simulink model "adjcochanint"  (Simulink 6.0)
settings: Solver=VariableStepDiscrete  SolverMode=SingleTasking  StartTime=0.0  StopTime=50000  RelTol=1e-3  AbsTol=1e-6
undefined symbols (not defined in the file or in its folder): Fs, Rows, slcm, Tsym
libraries: dspsrcs4 x8, simulink x5, commdigbbndpm2 x4, dspsigattribs x4, commfilt2 x4, commrandsrc2 x3, commsink2 x2, dspsnks4 x2, dspmathops x2, commchan2 x1, dspsigops x1
CloseFcn:
  | clear adjcoSigsOut
settings Model: RequirementInfo=9  CovMetricSettings=d  Creator=tdelve  LastModifiedBy=arodrigu  ExtModeTrigMode=oneshot  ExtModeArmWhenConnect=off  ExtModeAutoUpdateStatusClock=off  ProdHWDeviceType=Specified
settings DataIOCC: LimitDataPoints=off  SaveOutput=off  SaveTime=off  SignalLoggingName=adjcoSigsOut
settings OptimizationCC: BlockReduction=off  BooleanDataType=off
settings DebuggingCC: CheckExecutionContextPreStartOutputMsg=on  CheckExecutionContextRuntimeOutputMsg=on  SolverPrmCheckMsg=none  InheritedTsInSrcMsg=none  IntegerOverflowMsg=none
settings HardwareCC: ProdHWDeviceType=Specified
settings ModelReferenceCC: UpdateModelReferenceTargets=IfOutOfDate
settings CodeAppCC: MangleLength=5

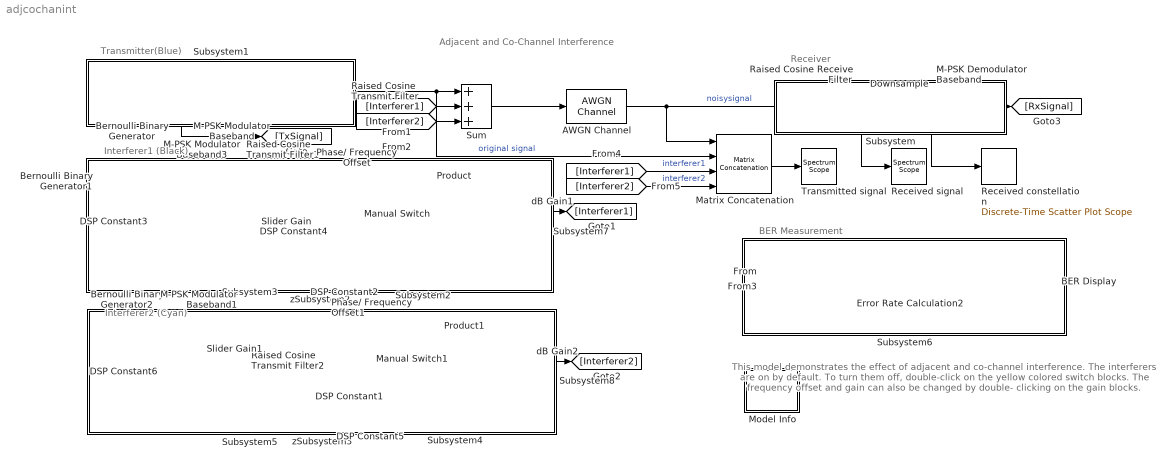
== system adjcochanint ==
  note: Adjacent and Co-Channel Interference
  note: Interferer1 (Black)
  note: Transmitter(Blue)
  note: Interferer2 (Cyan)
  note: Receiver
  note: BER Measurement
  note: This model demonstrates the effect of adjacent
      | and co-channel interference. The interferers are
      | on by default. To turn them off, double-click on
      | the yellow colored switch blocks. The frequency
      | offset and gain can also be changed by double-
      | clicking on the gain blocks.
  AWGN Channel : commchan2/AWGN Channel  seed=123456  noiseMode="Signal to noise ratio  (Es/No)"  EbNodB=10  EsNodB=30  SNRdB=10  bitsPerSym=1  Ps=1/8  Tsym=1e-6  variance=1
  BER Display : Display
  Bernoulli Binary Generator : commrandsrc2/Bernoulli Binary Generator  P=0.5  seed=529558  Ts=1e-6/3  frameBased=on  sampPerFrame=300  orient=off
  Bernoulli Binary Generator1 : commrandsrc2/Bernoulli Binary Generator  P=0.5  seed=529573  Ts=1e-6/3  frameBased=on  sampPerFrame=300  orient=off
  Bernoulli Binary Generator2 : commrandsrc2/Bernoulli Binary Generator  P=0.5  seed=529397  Ts=1e-6/3  frameBased=on  sampPerFrame=300  orient=off
  DSP Constant1 : dspsrcs4/DSP Constant  Value=0  SampleMode=Discrete  discreteOutput=Frame-based  continuousOutput=Sample-based  sampTime=Tsym*300  framePeriod=(1e-6/3)*300  dataType=Inherit from 'Constant value'  isSigned=on  wordLen=16  udDataType=sfix(16)  fracBitsMode=Best precision  numFracBits=15  InterpretAs1D=-inf  Ts=-inf  FramebasedOutput=-inf
  DSP Constant2 : dspsrcs4/DSP Constant  Value=1  SampleMode=Discrete  discreteOutput=Frame-based  continuousOutput=Sample-based  sampTime=Tsym*300  framePeriod=(1e-6/3)*300  dataType=Inherit from 'Constant value'  isSigned=on  wordLen=16  udDataType=sfix(16)  fracBitsMode=Best precision  numFracBits=15  InterpretAs1D=-inf  Ts=-inf  FramebasedOutput=-inf
  DSP Constant3 : dspsrcs4/DSP Constant  Value=-4e6  SampleMode=Discrete  discreteOutput=Frame-based  continuousOutput=Sample-based  sampTime=Tsym*100  framePeriod=(1e-6/3)*300  dataType=Inherit from 'Constant value'  isSigned=on  wordLen=16  udDataType=sfix(16)  fracBitsMode=Best precision  numFracBits=15  InterpretAs1D=-inf  Ts=-inf  FramebasedOutput=-inf
  DSP Constant4 : dspsrcs4/DSP Constant  Value=0  SampleMode=Discrete  discreteOutput=Frame-based  continuousOutput=Sample-based  sampTime=Tsym*300  framePeriod=(1e-6/3)*300  dataType=Inherit from 'Constant value'  isSigned=on  wordLen=16  udDataType=sfix(16)  fracBitsMode=Best precision  numFracBits=15  InterpretAs1D=-inf  Ts=-inf  FramebasedOutput=-inf
  DSP Constant5 : dspsrcs4/DSP Constant  Value=1  SampleMode=Discrete  discreteOutput=Frame-based  continuousOutput=Sample-based  sampTime=Tsym*300  framePeriod=(1e-6/3)*300  dataType=Inherit from 'Constant value'  isSigned=on  wordLen=16  udDataType=sfix(16)  fracBitsMode=Best precision  numFracBits=15  InterpretAs1D=-inf  Ts=-inf  FramebasedOutput=-inf
  DSP Constant6 : dspsrcs4/DSP Constant  Value=4e6  SampleMode=Discrete  discreteOutput=Frame-based  continuousOutput=Sample-based  sampTime=Tsym*300  framePeriod=(1e-6/3)*300  dataType=Inherit from 'Constant value'  isSigned=on  wordLen=16  udDataType=sfix(16)  fracBitsMode=Best precision  numFracBits=15  InterpretAs1D=-inf  Ts=-inf  FramebasedOutput=-inf
  Downsample : dspsigops/Downsample  N=8  phase=0  ic=0  smode=Allow multirate  fmode=Maintain input frame rate
  Error Rate Calculation2 : commsink2/Error Rate Calculation  N=12*3  st_delay=0  cp_mode=Entire frame  subframe=[]  PMode=Port  WsName=e1  RsMode2=off  stop=off  numErr=100  maxBits=1e6
  M-PSK Demodulator Baseband : commdigbbndpm2/M-PSK Demodulator Baseband  M=8  OutType=Bit  Dec=Gray  Ph=0  numSamp=1
  M-PSK Modulator Baseband : commdigbbndpm2/M-PSK Modulator Baseband  M=8  InType=Bit  Enc=Gray  Ph=0  numSamp=1
  M-PSK Modulator Baseband1 : commdigbbndpm2/M-PSK Modulator Baseband  M=8  InType=Bit  Enc=Gray  Ph=0  numSamp=1
  M-PSK Modulator Baseband3 : commdigbbndpm2/M-PSK Modulator Baseband  M=8  InType=Bit  Enc=Gray  Ph=0  numSamp=1
  Manual Switch : simulink/Signal Routing/Manual Switch  sw=0  action=0
  Manual Switch1 : simulink/Signal Routing/Manual Switch  sw=0  action=0
  Matrix Concatenation : simulink/Math Operations/Matrix Concatenation  numInports=4  catMethod=Horizontal
  Model Info : Subsystem  LoadFcn=slcm LoadBlock;  InitFcn=slcm('UpdateAllCMBlocksInThisModelInit')  PropExecContextAcrossSSBoundary=on  mask(CMBlock){InitialSaveTempField=, InitialBlockCM=none, BlockCM=none, Frame=on, SaveTempField=, DisplayStringWithTags=Info, MaskDisplayString=Info, HorizontalTextAlignment=Center, LeftAlignmentValue=0.5, SourceBlockDiagram=adjcochanint, TagMaxNumber=20, CMTag1=, CMTag2=, CMTag3=, CMTag4=, CMTag5=, CMTag6=, CMTag7=, CMTag8=, CMTag9=, CMTag10=, CMTag11=, CMTag12=, CMTag13=, CMTag14=, CMTag15=, CMTag16=, CMTag17=, CMTag18=, CMTag19=, CMTag20=}
      mask help: This block allows revision control information to be displayed within the model.
      settings: CopyFcn=slcm CopyBlock;  DeleteFcn=slcm Cancel;  PostSaveFcn=slcm('UpdateAllCMBlocksInThisModel')  NameChangeFcn=slcm Rename;  OpenFcn=commdemohelp;
      mask Display: text(str2num(LeftAlignmentValue), 0.5, MaskDisplayString, 'HorizontalAlignment', HorizontalTextAlignment)
  Phase/ Frequency Offset : Subsystem  PropExecContextAcrossSSBoundary=on  mask(Phase/Frequency Offset){phaseOffset=0}
      mask prompts: phaseOffset "Phase offset (deg):"
      mask help: Complex baseband model of residual phase and frequency offsets.
      mask Help: helpview(commbhelp)
      mask Display: disp('Phase/\nFrequency\nOffset');
  Phase/ Frequency Offset1 : Subsystem  PropExecContextAcrossSSBoundary=on  mask(Phase/Frequency Offset){phaseOffset=0}
      mask prompts: phaseOffset "Phase offset (deg):"
      mask help: Complex baseband model of residual phase and frequency offsets.
      mask Help: helpview(commbhelp)
      mask Display: disp('Phase/\nFrequency\nOffset');
  Product : Product  SaturateOnIntegerOverflow=on
  Product1 : Product  SaturateOnIntegerOverflow=on
  Raised Cosine Receive Filter : commfilt2/Raised Cosine Receive Filter  filtType=Square root  N=8  D=6  R=0.22  sampMode=Frame-based  rateMode=None  downFactor=1  downOffset=0  checkGain=Normalized  filterGain=1  checkCoeff=off  variableName=rcRxFilt  launchFVT=off
  Raised Cosine Transmit Filter : commfilt2/Raised Cosine Transmit Filter  filtType=Square root  D=6  R=0.22  sampMode=Frame-based  N=8  checkGain=Normalized  filterGain=1  checkCoeff=off  variableName=rcTxFilt  launchFVT=off
  Raised Cosine Transmit Filter1 : commfilt2/Raised Cosine Transmit Filter  filtType=Square root  D=6  R=0.22  sampMode=Frame-based  N=8  checkGain=Normalized  filterGain=1  checkCoeff=off  variableName=rcTxFilt1  launchFVT=off
  Raised Cosine Transmit Filter2 : commfilt2/Raised Cosine Transmit Filter  filtType=Square root  D=6  R=0.22  sampMode=Frame-based  N=8  checkGain=Normalized  filterGain=1  checkCoeff=off  variableName=rcTxFilt2  launchFVT=off
  Received constellation : commsink2/Discrete-Time Scatter Plot Scope  Tag=ScatterPlot  sampPerSymb=1  offsetEye=0  numTraces=400  numNewFrames=100  LineMarkers=.  LineColors=b  fading=on  render=on  AxisGrid=on  xMin=-2.4831480177732  xMax=2.52514227621423  yMin=-2.47259861231716  yMax=2.53569168167027  inphaseLabel=In-phase Amplitude  quadratureLabel=Quadrature Amplitude  openScopeAtSimStart=on  FrameNumber=off  FigPos=[788 34 211 211]  figTitle=Scatter Plot  numLinesMax=8  block_type_=scatter
  Received signal : dspsnks4/Spectrum Scope  ScopeProperties=off  Domain=Frequency  HorizSpan=1  UseBuffer=on  BufferSize=128  Overlap=64  inpFftLenInherit=off  FFTlength=128  numAvg=10  DisplayProperties=on  AxisGrid=on  Memory=off  FrameNumber=off  AxisLegend=off  AxisZoom=off  OpenScopeAtSimStart=on  OpenScopeImmediately=off  FigPos=[381 47 357 145]  AxisProperties=off  XUnits=Hertz  XRange=[-Fs/2...Fs/2]  InheritXIncr=on  XIncr=1.0  XLabel=Samples  YUnits=dB  YLabel=Magnitude, dB  LineProperties=off  LineColors=[1 0 0]|[0 0 1]
      settings: YMin=-95.9893424566119  YMax=19.7294255518364
  Slider Gain : simulink/Math Operations/Slider Gain  low=0  gain=1  high=2
  Slider Gain1 : simulink/Math Operations/Slider Gain  low=0  gain=1.4  high=2
  Subsystem : Subsystem  Orientation=left  PropExecContextAcrossSSBoundary=on
      mask Display: disp('');
  Subsystem1 : Subsystem  Orientation=left  PropExecContextAcrossSSBoundary=on
      mask Display: disp('');
  Subsystem2 : Subsystem  Orientation=left  PropExecContextAcrossSSBoundary=on
      mask Display: disp('Double-click above\n to activate Interferer1');
  Subsystem3 : Subsystem  Orientation=left  PropExecContextAcrossSSBoundary=on
      mask Display: disp('Double-click above\n to change frequency offset');
  Subsystem4 : Subsystem  Orientation=left  PropExecContextAcrossSSBoundary=on
      mask Display: disp('Double-click above\n to activate Interferer2');
  Subsystem5 : Subsystem  Orientation=left  PropExecContextAcrossSSBoundary=on
      mask Display: disp('Double-click above\n to change frequency offset');
  Subsystem6 : Subsystem  Orientation=left  PropExecContextAcrossSSBoundary=on
      mask Display: disp('');
  Subsystem7 : Subsystem  Orientation=left  PropExecContextAcrossSSBoundary=on
      mask Display: disp('Double-click above\n to change gain');
  Subsystem8 : Subsystem  Orientation=left  PropExecContextAcrossSSBoundary=on
      mask Display: disp('Double-click above\n to change gain');
  Sum : Sum  Inputs=+++  SaturateOnIntegerOverflow=on
  Transmitted signal : dspsnks4/Spectrum Scope  ScopeProperties=off  Domain=Frequency  HorizSpan=1  UseBuffer=on  BufferSize=128  Overlap=64  inpFftLenInherit=off  FFTlength=128  numAvg=10  DisplayProperties=on  AxisGrid=on  Memory=off  FrameNumber=off  AxisLegend=off  AxisZoom=off  OpenScopeAtSimStart=on  OpenScopeImmediately=off  FigPos=[10 47 357 145]  AxisProperties=off  XUnits=Hertz  XRange=[-Fs/2...Fs/2]  InheritXIncr=on  XIncr=1.0  XLabel=Samples  YUnits=dB  YLabel=Magnitude, dB  LineProperties=off  LineColors=[1 0 0]|[0 0 1]|[0 0 0]|[0 1 1]
      settings: YMin=-91.8082302358486  YMax=10.0230122396749
  dB Gain1 : dspmathops/dB Gain  dB=-20  intype=Amplitude
  dB Gain2 : dspmathops/dB Gain  dB=-10  intype=Amplitude
  zSubsystem2 : Subsystem  Orientation=left  PropExecContextAcrossSSBoundary=on
      mask Display: disp('');
  zSubsystem3 : Subsystem  Orientation=left  PropExecContextAcrossSSBoundary=on
      mask Display: disp('');
  wires:
  M-PSK Modulator Baseband/1 -> Raised Cosine Transmit Filter/1
  Bernoulli Binary Generator1/1 -> M-PSK Modulator Baseband3/1
  M-PSK Modulator Baseband1/1 -> Raised Cosine Transmit Filter2/1
  M-PSK Modulator Baseband3/1 -> Raised Cosine Transmit Filter1/1
  Raised Cosine Transmit Filter1/1 -> Phase/ Frequency Offset/1(In)
  Raised Cosine Transmit Filter2/1 -> Phase/ Frequency Offset1/1(In)
  Raised Cosine Transmit Filter/1 -> Sum/1, Matrix Concatenation/2  "original signal"
  DSP Constant4/1 -> Manual Switch/1
  Manual Switch/1 -> Product/2
  DSP Constant2/1 -> Manual Switch/2
  DSP Constant1/1 -> Manual Switch1/1
  Manual Switch1/1 -> Product1/2
  DSP Constant5/1 -> Manual Switch1/2
  Phase/ Frequency Offset1/1(Out) -> Product1/1
  Slider Gain/1 -> Phase/ Frequency Offset/2(In1)
  DSP Constant3/1 -> Slider Gain/1
  DSP Constant6/1 -> Slider Gain1/1
  Slider Gain1/1 -> Phase/ Frequency Offset1/2(In1)
  Bernoulli Binary Generator/1 -> M-PSK Modulator Baseband/1, [TxSignal]
  Bernoulli Binary Generator2/1 -> M-PSK Modulator Baseband1/1
  Phase/ Frequency Offset/1(Out) -> Product/1
  Sum/1 -> AWGN Channel/1
  AWGN Channel/1 -> Raised Cosine Receive Filter/1, Matrix Concatenation/1  "noisysignal"
  Raised Cosine Receive Filter/1 -> Received signal/1, Downsample/1
  Downsample/1 -> Received constellation/1, M-PSK Demodulator Baseband/1
  M-PSK Demodulator Baseband/1 -> [RxSignal]
  Product/1 -> dB Gain1/1
  Product1/1 -> dB Gain2/1
  [Interferer1] -> Sum/2
  [Interferer2] -> Sum/3
  Matrix Concatenation/1 -> Transmitted signal/1
  [TxSignal] -> Error Rate Calculation2/1
  [RxSignal] -> Error Rate Calculation2/2
  dB Gain1/1 -> [Interferer1]
  dB Gain2/1 -> [Interferer2]
  [Interferer1] -> Matrix Concatenation/3  "interferer1"
  [Interferer2] -> Matrix Concatenation/4  "interferer2"
  Error Rate Calculation2/1 -> BER Display/1

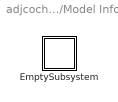
== system adjcochanint/Model Info ==
  EmptySubsystem : Subsystem  PropExecContextAcrossSSBoundary=on

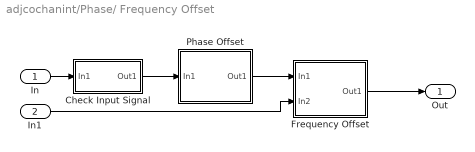
== system adjcochanint/Phase/ Frequency Offset ==
  In : Inport  LatchInput=off
  In1 : Inport  Port=2  LatchInput=off
  Check Input Signal : Subsystem  PropExecContextAcrossSSBoundary=on
      mask Display: disp('Check\nInput Signal');
  Frequency Offset : Subsystem  PropExecContextAcrossSSBoundary=on
      mask Display: disp('Frequency\nOffset');
  Phase Offset : Subsystem  PropExecContextAcrossSSBoundary=on
      mask Display: disp('Phase\nOffset');
  Out : Outport
  wires:
  Check Input Signal/1(Out1) -> Phase Offset/1(In1)
  Phase Offset/1(Out1) -> Frequency Offset/1(In1)
  In/1 -> Check Input Signal/1(In1)
  Frequency Offset/1(Out1) -> Out/1
  In1/1 -> Frequency Offset/2(In2)

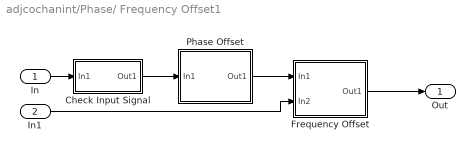
== system adjcochanint/Phase/ Frequency Offset1 ==
  In : Inport  LatchInput=off
  In1 : Inport  Port=2  LatchInput=off
  Check Input Signal : Subsystem  PropExecContextAcrossSSBoundary=on
      mask Display: disp('Check\nInput Signal');
  Frequency Offset : Subsystem  PropExecContextAcrossSSBoundary=on
      mask Display: disp('Frequency\nOffset');
  Phase Offset : Subsystem  PropExecContextAcrossSSBoundary=on
      mask Display: disp('Phase\nOffset');
  Out : Outport
  wires:
  In1/1 -> Frequency Offset/2(In2)
  Frequency Offset/1(Out1) -> Out/1
  In/1 -> Check Input Signal/1(In1)
  Phase Offset/1(Out1) -> Frequency Offset/1(In1)
  Check Input Signal/1(Out1) -> Phase Offset/1(In1)

== system adjcochanint/Subsystem ==

== system adjcochanint/Subsystem1 ==

== system adjcochanint/Subsystem2 ==

== system adjcochanint/Subsystem3 ==

== system adjcochanint/Subsystem4 ==

== system adjcochanint/Subsystem5 ==

== system adjcochanint/Subsystem6 ==

== system adjcochanint/Subsystem7 ==

== system adjcochanint/Subsystem8 ==

== system adjcochanint/zSubsystem2 ==

== system adjcochanint/zSubsystem3 ==

== system adjcochanint/Model Info/EmptySubsystem ==

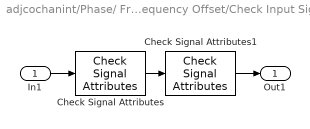
== system adjcochanint/Phase/ Frequency Offset/Check Input Signal ==
  In1 : Inport  LatchInput=off
  Check Signal Attributes : dspsigattribs/Check Signal Attributes  SigAttribCheckMethod=Does not match attributes exactly  Complexity=Complex  Frame=Ignore  DimsCheckMethod=Is...  Dimensions=Column vector (2-D) or scalar  DatatypeCheckMethod=Ignore  DatatypeGeneral=Boolean  DtypeFloatSpecific=Any floating-point  DtypeFixedSpecific=Any fixed-point  DtypeIntSpecific=Any integer  SampleMode=Ignore
  Check Signal Attributes1 : dspsigattribs/Check Signal Attributes  SigAttribCheckMethod=Matches attributes exactly  Complexity=Ignore  Frame=Sample-based  DimsCheckMethod=Is...  Dimensions=Vector (1-D or 2-D)  DatatypeCheckMethod=Ignore  DatatypeGeneral=Boolean  DtypeFloatSpecific=Any floating-point  DtypeFixedSpecific=Any fixed-point  DtypeIntSpecific=Any integer  SampleMode=Ignore
  Out1 : Outport
  wires:
  In1/1 -> Check Signal Attributes/1
  Check Signal Attributes1/1 -> Out1/1
  Check Signal Attributes/1 -> Check Signal Attributes1/1

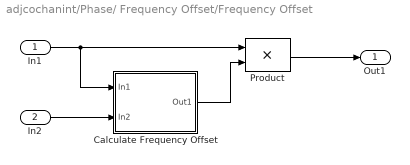
== system adjcochanint/Phase/ Frequency Offset/Frequency Offset ==
  In1 : Inport  LatchInput=off
  In2 : Inport  Port=2  LatchInput=off
  Calculate Frequency Offset : Subsystem  PropExecContextAcrossSSBoundary=on
      mask Display: disp('Calculate\nFrequency\nOffset');
  Product : Product  SaturateOnIntegerOverflow=on  InputSameDT=on
  Out1 : Outport
  wires:
  Calculate Frequency Offset/1(Out1) -> Product/2
  In1/1 -> Calculate Frequency Offset/1(In1), Product/1
  Product/1 -> Out1/1
  In2/1 -> Calculate Frequency Offset/2(In2)

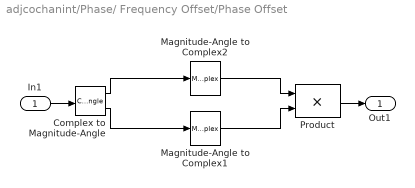
== system adjcochanint/Phase/ Frequency Offset/Phase Offset ==
  In1 : Inport  LatchInput=off
  Complex to Magnitude-Angle : ComplexToMagnitudeAngle
  Magnitude-Angle to Complex1 : MagnitudeAngleToComplex  Input=Angle  ConstantPart=1
  Magnitude-Angle to Complex2 : MagnitudeAngleToComplex  Input=Magnitude  ConstantPart=phaseOffset*pi/180
  Product : Product  SaturateOnIntegerOverflow=on  InputSameDT=on
  Out1 : Outport
  wires:
  Product/1 -> Out1/1
  In1/1 -> Complex to Magnitude-Angle/1
  Magnitude-Angle to Complex1/1 -> Product/2
  Magnitude-Angle to Complex2/1 -> Product/1
  Complex to Magnitude-Angle/1 -> Magnitude-Angle to Complex2/1
  Complex to Magnitude-Angle/2 -> Magnitude-Angle to Complex1/1

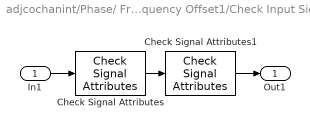
== system adjcochanint/Phase/ Frequency Offset1/Check Input Signal ==
  In1 : Inport  LatchInput=off
  Check Signal Attributes : dspsigattribs/Check Signal Attributes  SigAttribCheckMethod=Does not match attributes exactly  Complexity=Complex  Frame=Ignore  DimsCheckMethod=Is...  Dimensions=Column vector (2-D) or scalar  DatatypeCheckMethod=Ignore  DatatypeGeneral=Boolean  DtypeFloatSpecific=Any floating-point  DtypeFixedSpecific=Any fixed-point  DtypeIntSpecific=Any integer  SampleMode=Ignore
  Check Signal Attributes1 : dspsigattribs/Check Signal Attributes  SigAttribCheckMethod=Matches attributes exactly  Complexity=Ignore  Frame=Sample-based  DimsCheckMethod=Is...  Dimensions=Vector (1-D or 2-D)  DatatypeCheckMethod=Ignore  DatatypeGeneral=Boolean  DtypeFloatSpecific=Any floating-point  DtypeFixedSpecific=Any fixed-point  DtypeIntSpecific=Any integer  SampleMode=Ignore
  Out1 : Outport
  wires:
  Check Signal Attributes/1 -> Check Signal Attributes1/1
  Check Signal Attributes1/1 -> Out1/1
  In1/1 -> Check Signal Attributes/1

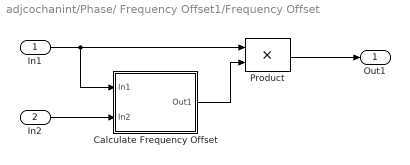
== system adjcochanint/Phase/ Frequency Offset1/Frequency Offset ==
  In1 : Inport  LatchInput=off
  In2 : Inport  Port=2  LatchInput=off
  Calculate Frequency Offset : Subsystem  PropExecContextAcrossSSBoundary=on
      mask Display: disp('Calculate\nFrequency\nOffset');
  Product : Product  SaturateOnIntegerOverflow=on  InputSameDT=on
  Out1 : Outport
  wires:
  In2/1 -> Calculate Frequency Offset/2(In2)
  Product/1 -> Out1/1
  In1/1 -> Product/1, Calculate Frequency Offset/1(In1)
  Calculate Frequency Offset/1(Out1) -> Product/2

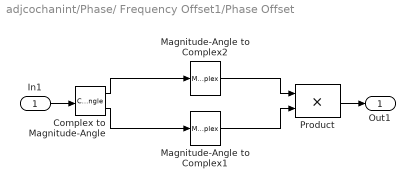
== system adjcochanint/Phase/ Frequency Offset1/Phase Offset ==
  In1 : Inport  LatchInput=off
  Complex to Magnitude-Angle : ComplexToMagnitudeAngle
  Magnitude-Angle to Complex1 : MagnitudeAngleToComplex  Input=Angle  ConstantPart=1
  Magnitude-Angle to Complex2 : MagnitudeAngleToComplex  Input=Magnitude  ConstantPart=phaseOffset*pi/180
  Product : Product  SaturateOnIntegerOverflow=on  InputSameDT=on
  Out1 : Outport
  wires:
  Complex to Magnitude-Angle/2 -> Magnitude-Angle to Complex1/1
  Complex to Magnitude-Angle/1 -> Magnitude-Angle to Complex2/1
  Magnitude-Angle to Complex2/1 -> Product/1
  Magnitude-Angle to Complex1/1 -> Product/2
  In1/1 -> Complex to Magnitude-Angle/1
  Product/1 -> Out1/1

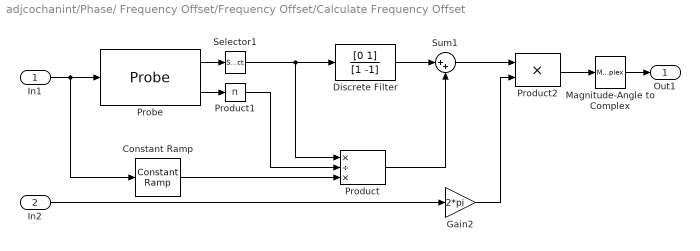
== system adjcochanint/Phase/ Frequency Offset/Frequency Offset/Calculate Frequency Offset ==
  In1 : Inport  LatchInput=off
  In2 : Inport  Port=2  LatchInput=off
  Constant Ramp : dspsrcs4/Constant Ramp  L=Rows  Slope=1  dataType=Same as input  wordLen=16  udDataType=sfix(16)  fracBitsMode=Best precision  numFracBits=15  Offset=0
  Discrete Filter : DiscreteFilter  Numerator=[0 1]  Denominator=[1 -1]  SampleTime=-1
  Gain2 : Gain  Gain=2*pi  SaturateOnIntegerOverflow=on
  Magnitude-Angle to Complex : MagnitudeAngleToComplex  Input=Angle  ConstantPart=1
  Probe : Probe  ProbeWidth=off  ProbeComplexSignal=off  ProbeSignalDimensions=on
  Product : Product  Inputs=*/*  SaturateOnIntegerOverflow=on  InputSameDT=on
  Product1 : Product  Inputs=1  SaturateOnIntegerOverflow=on  InputSameDT=on
  Product2 : Product  SaturateOnIntegerOverflow=on
  Selector1 : Selector  Elements=[1 ]  InputPortWidth=2
  Sum1 : Sum  Inputs=|++  SaturateOnIntegerOverflow=on  InputSameDT=on
  Out1 : Outport
  wires:
  Selector1/1 -> Discrete Filter/1, Product/1
  Discrete Filter/1 -> Sum1/1
  Product1/1 -> Product/2
  Product2/1 -> Magnitude-Angle to Complex/1
  Sum1/1 -> Product2/1
  Constant Ramp/1 -> Product/3
  Probe/1 -> Selector1/1
  Product/1 -> Sum1/2
  Probe/2 -> Product1/1
  In1/1 -> Constant Ramp/1, Probe/1
  Magnitude-Angle to Complex/1 -> Out1/1
  In2/1 -> Gain2/1
  Gain2/1 -> Product2/2

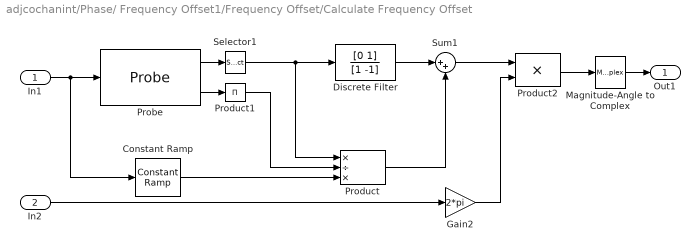
== system adjcochanint/Phase/ Frequency Offset1/Frequency Offset/Calculate Frequency Offset ==
  In1 : Inport  LatchInput=off
  In2 : Inport  Port=2  LatchInput=off
  Constant Ramp : dspsrcs4/Constant Ramp  L=Rows  Slope=1  dataType=Same as input  wordLen=16  udDataType=sfix(16)  fracBitsMode=Best precision  numFracBits=15  Offset=0
  Discrete Filter : DiscreteFilter  Numerator=[0 1]  Denominator=[1 -1]  SampleTime=-1
  Gain2 : Gain  Gain=2*pi  SaturateOnIntegerOverflow=on
  Magnitude-Angle to Complex : MagnitudeAngleToComplex  Input=Angle  ConstantPart=1
  Probe : Probe  ProbeWidth=off  ProbeComplexSignal=off  ProbeSignalDimensions=on
  Product : Product  Inputs=*/*  SaturateOnIntegerOverflow=on  InputSameDT=on
  Product1 : Product  Inputs=1  SaturateOnIntegerOverflow=on  InputSameDT=on
  Product2 : Product  SaturateOnIntegerOverflow=on
  Selector1 : Selector  Elements=[1 ]  InputPortWidth=2
  Sum1 : Sum  Inputs=|++  SaturateOnIntegerOverflow=on  InputSameDT=on
  Out1 : Outport
  wires:
  Gain2/1 -> Product2/2
  In2/1 -> Gain2/1
  Magnitude-Angle to Complex/1 -> Out1/1
  In1/1 -> Probe/1, Constant Ramp/1
  Probe/2 -> Product1/1
  Product/1 -> Sum1/2
  Probe/1 -> Selector1/1
  Constant Ramp/1 -> Product/3
  Sum1/1 -> Product2/1
  Product2/1 -> Magnitude-Angle to Complex/1
  Product1/1 -> Product/2
  Discrete Filter/1 -> Sum1/1
  Selector1/1 -> Product/1, Discrete Filter/1
